simulink model "RL_comp3"  (R2017a)
settings: Solver=VariableStepAuto  StartTime=0.0  StopTime=10.0  RelTol=1e-3
libraries: dspsigops x2
settings Model: Creator=venkat  LastModifiedBy=venkat

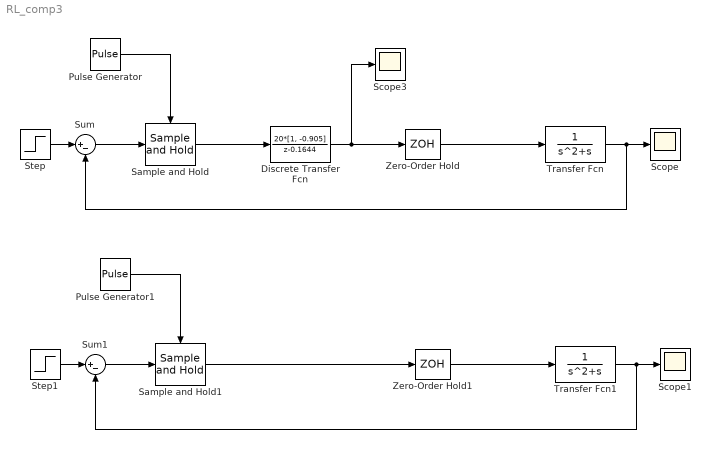
== system RL_comp3 ==
  Discrete Transfer Fcn : DiscreteTransferFcn  Numerator=20*[1, -0.905]  Denominator=[1, -0.1644]  SampleTime=0.1
  Pulse Generator : DiscretePulseGenerator  PulseType=Time based  Period=0.1  PulseWidth=5
  Pulse Generator1 : DiscretePulseGenerator  PulseType=Time based  Period=0.1  PulseWidth=5
  Sample and Hold : dspsigops/Sample and Hold  trig=Rising edge  initCond=0  latchinput=off
  Sample and Hold1 : dspsigops/Sample and Hold  trig=Rising edge  initCond=0  latchinput=off
  Scope : Scope
  Scope1 : Scope
  Scope3 : Scope
  Step : Step  SampleTime=0
  Step1 : Step  SampleTime=0
  Sum : Sum  Inputs=|+-
  Sum1 : Sum  Inputs=|+-
  Transfer Fcn : TransferFcn  Denominator=[1 1 0]
  Transfer Fcn1 : TransferFcn  Denominator=[1 1 0]
  Zero-Order Hold : ZeroOrderHold  SampleTime=-1
  Zero-Order Hold1 : ZeroOrderHold  SampleTime=-1
  wires:
  Step/1 -> Sum/1
  Pulse Generator/1 -> Sample and Hold/Trigger
  Sum/1 -> Sample and Hold/1
  Sample and Hold/1 -> Discrete Transfer Fcn/1
  Zero-Order Hold/1 -> Transfer Fcn/1
  Transfer Fcn/1 -> Sum/2, Scope/1
  Transfer Fcn1/1 -> Sum1/2, Scope1/1
  Zero-Order Hold1/1 -> Transfer Fcn1/1
  Sum1/1 -> Sample and Hold1/1
  Step1/1 -> Sum1/1
  Sample and Hold1/1 -> Zero-Order Hold1/1
  Pulse Generator1/1 -> Sample and Hold1/Trigger
  Discrete Transfer Fcn/1 -> Scope3/1, Zero-Order Hold/1
